simulink model "Cinco_Gunay_Laboratory_No_3"  (R2023b)
settings: Solver=VariableStepAuto  StartTime=0.0  StopTime=20.0  RelTol=1e-3
values from neighbouring files (symbols this model uses):
  G_den = [1 -2 2 -1 -2 2 1 -1 0 0 0]    [Cinco_Gunay_Lab_No_3.m]    (also in Dela_Roca_Dipasupil_Lab_No_3.m = [4 -8 -4 14 -8 -2 2 6 4 0 0 0 0])
  G_num = [1 2]    [Cinco_Gunay_Lab_No_3.m]    (also in Dela_Roca_Dipasupil_Lab_No_3.m = [2 -6 4 0 0 0 0 0])
settings Model: Creator=Ian Gunay  LastModifiedBy=Ian Gunay

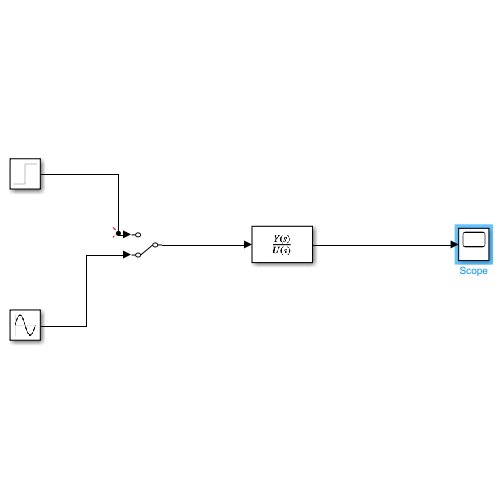
[thumbnail: Simulink's stored preview of the top-level diagram]
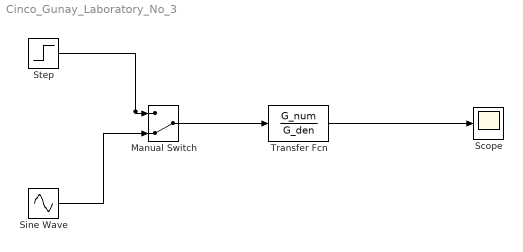
== system Cinco_Gunay_Laboratory_No_3 ==
  Manual Switch : ManualSwitch  CurrentSetting=0
  Scope : Scope
  Sine Wave : Sin  SampleTime=0
  Step : Step  SampleTime=0
  Transfer Fcn : TransferFcn  Numerator=G_num  Denominator=G_den
  wires:
  Sine Wave/1 -> Manual Switch/2
  Transfer Fcn/1 -> Scope/1
  Manual Switch/1 -> Transfer Fcn/1
  Step/1 -> Manual Switch/1
